simulink model "PID_C"  (R2020b)
settings: Solver=VariableStepAuto  StartTime=0.0  StopTime=120  RelTol=1e-3
model workspace (MAT data in the model file):
  Kd = Simulink.Parameter
  Kd.Value = 0
  Kd.DataType = 'auto'
  Kd.Dimensions = [1 1]
  Ki = Simulink.Parameter
  Ki.Value = 90
  Ki.DataType = 'auto'
  Ki.Dimensions = [1 1]
  Kp = Simulink.Parameter
  Kp.Value = 550
  Kp.DataType = 'auto'
  Kp.Dimensions = [1 1]
values from neighbouring files (symbols this model uses):
  Kd = 0.0    [Data.sldd]
  Ki = 90.0    [Data.sldd]
  Kp = 550.0    [Data.sldd]
settings Model: DataDictionary=Data.sldd  Creator=smart  LastModifiedBy=smart
settings DataIOCC: SaveOutput=off  SaveTime=off

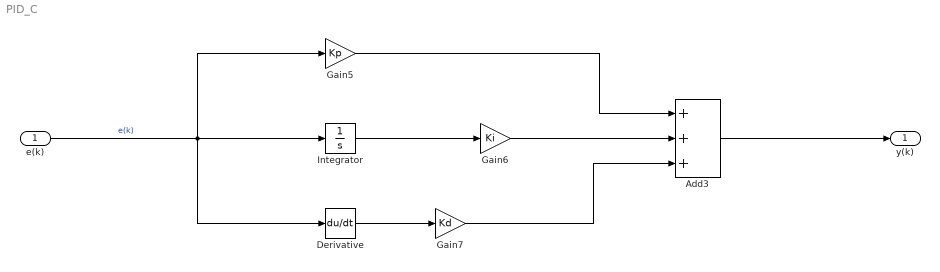
== system PID_C ==
  e(k) : Inport  OutDataTypeStr=double  PortDimensions=1  SampleTime=0
  Add3 : Sum  Inputs=+++
  Derivative : Derivative
  Gain5 : Gain  Gain=Kp
  Gain6 : Gain  Gain=Ki
  Gain7 : Gain  Gain=Kd
  Integrator : Integrator
  y(k) : Outport  OutDataTypeStr=double  PortDimensions=1  SampleTime=0
  wires:
  Derivative/1 -> Gain7/1
  Add3/1 -> y(k)/1
  Gain6/1 -> Add3/2
  Integrator/1 -> Gain6/1
  Gain7/1 -> Add3/3
  e(k)/1 -> Gain5/1, Integrator/1, Derivative/1  "e(k)"
  Gain5/1 -> Add3/1
